simulink model "KalmanIMU"  (R2018a)
settings: Solver=VariableStepAuto  StartTime=0.0  StopTime=10.0  RelTol=1e-3
settings Model: Creator=55119  LastModifiedBy=gmore

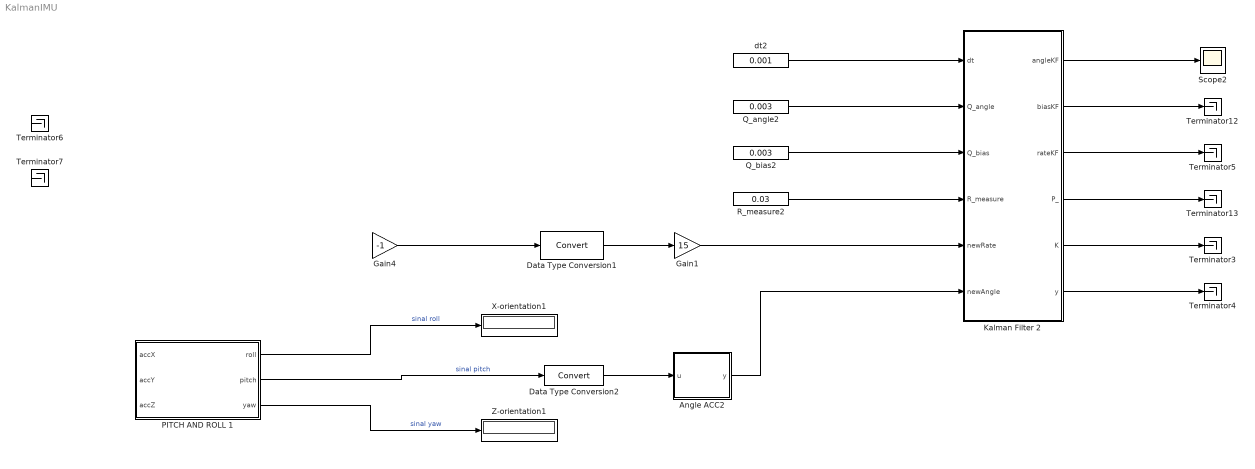
== system KalmanIMU ==
  Angle ACC2 : MATLAB Function  TreatAsAtomicUnit=on
  Data Type Conversion1 : DataTypeConversion
  Data Type Conversion2 : DataTypeConversion
  Gain1 : Gain  Gain=15
  Gain4 : Gain  Gain=-1
  Kalman Filter 2 : MATLAB Function  TreatAsAtomicUnit=on
  PITCH AND ROLL 1 : MATLAB Function  TreatAsAtomicUnit=on
  Q_angle2 : Constant  Value=0.003
  Q_bias2 : Constant  Value=0.003
  R_measure2 : Constant  Value=0.03
  Scope2 : Scope
  Terminator{3..7,12..13} (7 alike) : Terminator
  X-orientation1 : Display
      settings: Format=bank
  Z-orientation1 : Display
      settings: Format=bank
  dt2 : Constant  Value=0.001
  wires:
  ? -> Terminator6/1  "<q>"
  ? -> PITCH AND ROLL 1/2(accY)  "<ddy>"
  ? -> PITCH AND ROLL 1/1(accX)  "<ddx>"
  ? -> PITCH AND ROLL 1/3(accZ)  "<ddz>"
  ? -> Gain4/1  "<p>"
  ? -> Terminator7/1  "<r>"
  Kalman Filter 2/2(biasKF) -> Terminator12/1
  Data Type Conversion2/1 -> Angle ACC2/1(u)
  PITCH AND ROLL 1/3(yaw) -> Z-orientation1/1  "sinal yaw"
  dt2/1 -> Kalman Filter 2/1(dt)
  Kalman Filter 2/3(rateKF) -> Terminator5/1
  PITCH AND ROLL 1/2(pitch) -> Data Type Conversion2/1  "sinal pitch"
  Kalman Filter 2/6(y) -> Terminator4/1
  Angle ACC2/1(y) -> Kalman Filter 2/6(newAngle)
  Q_angle2/1 -> Kalman Filter 2/2(Q_angle)
  Gain1/1 -> Kalman Filter 2/5(newRate)
  Kalman Filter 2/1(angleKF) -> Scope2/1
  Kalman Filter 2/4(P_) -> Terminator13/1
  Kalman Filter 2/5(K) -> Terminator3/1
  Gain4/1 -> Data Type Conversion1/1
  Data Type Conversion1/1 -> Gain1/1
  R_measure2/1 -> Kalman Filter 2/4(R_measure)
  PITCH AND ROLL 1/1(roll) -> X-orientation1/1  "sinal roll"
  Q_bias2/1 -> Kalman Filter 2/3(Q_bias)

== matlab function KalmanIMU/Angle ACC2 ==
  data: u input; y output
function y = fcn(u)

if(isnan(u))
y=0;
else
y=u;
end

== matlab function KalmanIMU/Kalman Filter 2 ==
  data: angleKF output; biasKF output; rateKF output; dt input; Q_angle input; Q_bias input; R_measure input; newRate input; newAngle input; P_ output; K output; y output
%guilherme moreira rodrigues UFPB 20160105205
function [angleKF, biasKF, rateKF, P_, K, y] = fcn(dt, Q_angle, Q_bias, R_measure, newRate, newAngle)


%matriz de covariância de erro (ruido de processo)
Q = [Q_angle 0;0 Q_bias]*dt;
A = [1  -dt;0  1];
C = [1 0];

angleKF = 0.0; %Redefine angulo
biasKF = 0.0;  %Redefine bias

%Equações discretas de atualização do tempo do filtro de kalman (projeta o estado a frente)
rateKF = newRate - biasKF;

persistent angle;
if isempty(angle)
angle = 0;
else angle = angle + (dt * rateKF); 
end
angleKF = angle;

%atualiza a matriz de covariancia da estimativa de erro (projeta a covariancia de erro do estado a frente)
persistent P;
if isempty(P);P = [0 0 ; 0 0]; 
else P = A*P*A' + Q;
end
P_ = P

%equações discretas de atualização de medição do filtro de kalman (Calcula o ganho de kalman)
S = C*P*C' + R_measure; %estimativa de erro
K = (P_*C')/S %ganho de kalman 

%calcular a estimativa do novo angulo
y = newAngle - angleKF; %diferença de angulo
xk = angleKF + K*y
angleKF = xk(1);
biasKF = xk(2);
angle = angleKF

%atualizar a covariancia de erro
I = [1 0;0 1];
P_ = (I - K*C)*P_;

P = P_;

return

end

== matlab function KalmanIMU/PITCH AND ROLL 1 ==
  data: accX input; roll output; pitch output; yaw output; accY input; accZ input

function [roll,...
          pitch,...
          yaw]...
          = OrientationFcn(accX, accY, accZ)
    
X2 = rad2deg(accX);
Y2 = rad2deg(accY);
Z3 = rad2deg(accZ);

roll = atan2(Y2, Z3);

pitch = atan2(-X2, sqrt(Y2*Y2 + Z3*Z3));

yaw = Z3; 
   
      
      
      
      
      
      
      
      
end
